simulink model "BG"  (R2014a)
settings: Solver=ode3  StartTime=0.0  StopTime=1  FixedStep=dt  MaxStep=dt  RelTol=1e-3
values from neighbouring files (symbols this model uses):
  a1 = .4    (= 0.4)    [parameters.m]
  a2 = .35    (= 0.35)    [parameters.m]
  a3 = .25    (= 0.25)    [parameters.m]
  aTc = 0.05    [parameters.m]
  dt = 1e-3    (= 0.001)    [parameters.m]
  g = 1    [parameters.m]
  K = 1    [parameters.m]
  mTc = 0.01    [parameters.m]
  OP1_0 = [ax1_0 ay1_0 0]    [parameters.m]
  OP2_0 = OP1_0 + P1P2_0    [parameters.m]
  OP3_0 = OP2_0 + P2P3_0    [parameters.m]
  OT = [xf yf 0]    [animation.m]    (also in parameters.m = [0.5 0.5 0])
  OT_cercle = [0.6 0.55 0]    [parameters.m]
  p1 = w2 + w3    (= 3)    [parameters.m]
  P1P2_0 = [ax2_0 ay2_0 0]    [parameters.m]
  p2 = w1 + w3    (= 4)    [parameters.m]
  P2P3_0 = [ax3_0 ay3_0 0]    [parameters.m]
  p3 = w2 + w1    (= 5)    [parameters.m]
  tau = 0.001    [parameters.m]
  theta1_0 = zero_vector    [parameters.m]
  theta2_0 = zero_vector    [parameters.m]
  theta3_0 = zero_vector    [parameters.m]
  Vmax = 30    [parameters.m]
  w1 = 3    [parameters.m]
  w2 = 2    [parameters.m]
  w3 = 1    [parameters.m]
  zero_vector = [0 0 0]    [parameters.m]
libraries: vrlib x9, simulink x1
(part 4 of 4)

== system BG/CNS/ Striosom//SNc2/Optimiseur/B2/Subsystem/matrix_by_matrix1 ==
  a11 : Inport
  a12 : Inport  Port=2
  a21 : Inport  Port=3
  a22 : Inport  Port=4
  b11 : Inport  Port=5
  b12 : Inport  Port=6
  b21 : Inport  Port=7
  b22 : Inport  Port=8
  "                                                                                                    " : Sum
  "                                                                                                     " : Sum
  "                                                                                                       " : Sum
  "                                                                                                          " : Sum
  a{1..8} (8 alike) : Product
  a11_out : Outport
  a12_out : Outport  Port=2
  a21_out : Outport  Port=3
  a22_out : Outport  Port=4
  wires:
  a11/1 -> a3/1, a1/1
  b11/1 -> a1/2, a5/2
  a12/1 -> a4/1, a2/1
  a1/1 -> "                                                                                                    "/1
  a2/1 -> "                                                                                                    "/2
  b21/1 -> a6/2, a2/2
  "                                                                                                    "/1 -> a11_out/1
  a3/1 -> "                                                                                                       "/1
  a4/1 -> "                                                                                                       "/2
  "                                                                                                       "/1 -> a12_out/1
  b22/1 -> a8/2, a4/2
  a21/1 -> a5/1, a7/1
  a5/1 -> "                                                                                                     "/1
  a6/1 -> "                                                                                                     "/2
  "                                                                                                     "/1 -> a21_out/1
  a7/1 -> "                                                                                                          "/1
  a8/1 -> "                                                                                                          "/2
  "                                                                                                          "/1 -> a22_out/1
  a22/1 -> a8/1, a6/1
  b12/1 -> a7/2, a3/2

== system BG/CNS/ Striosom//SNc2/Optimiseur/B2/Subsystem/vector_in_matrix_out1 ==
  v1 : Inport
  v2 : Inport  Port=2
  Demux : Demux  Outputs=3
  Demux1 : Demux  Outputs=3
  a{11..12,21..22} (4 alike) : Product
  a11_out : Outport
  a12_out : Outport  Port=2
  a21_out : Outport  Port=3
  a22_out : Outport  Port=4
  wires:
  v1/1 -> Demux/1
  v2/1 -> Demux1/1
  a11/1 -> a11_out/1
  Demux/1 -> a12/1, a11/1
  a12/1 -> a12_out/1
  a21/1 -> a21_out/1
  Demux/2 -> a22/1, a21/1
  a22/1 -> a22_out/1
  Demux1/1 -> a11/2, a21/2
  Demux1/2 -> a22/2, a12/2

== system BG/CNS/ Striosom//SNc2/Optimiseur/B2/Subsystem/vector_in_matrix_out2 ==
  v1 : Inport
  v2 : Inport  Port=2
  Demux : Demux  Outputs=3
  Demux1 : Demux  Outputs=3
  a{11..12,21..22} (4 alike) : Product
  a11_out : Outport
  a12_out : Outport  Port=2
  a21_out : Outport  Port=3
  a22_out : Outport  Port=4
  wires:
  v1/1 -> Demux/1
  v2/1 -> Demux1/1
  a11/1 -> a11_out/1
  Demux/1 -> a12/1, a11/1
  a12/1 -> a12_out/1
  a21/1 -> a21_out/1
  Demux/2 -> a22/1, a21/1
  a22/1 -> a22_out/1
  Demux1/1 -> a11/2, a21/2
  Demux1/2 -> a22/2, a12/2

== system BG/CNS/ Striosom//SNc2/Optimiseur/lambda/d=V^T(VV^T)^-1V/inverse_matrix ==
  a11 : Inport
  a12 : Inport  Port=2
  a21 : Inport  Port=3
  a22 : Inport  Port=4
  "                                                                                                    " : Sum  Inputs=+-+
  Divide{1..4} (4 alike) : Product  Inputs=*/
  Gain : Gain  Gain=-1
  Gain1 : Gain  Gain=-1
  a1 : Product
  a2 : Product
  eps : Constant  Value=1e-2
  a11_out : Outport
  a12_out : Outport  Port=2
  a21_out : Outport  Port=3
  a22_out : Outport  Port=4
  wires:
  a11/1 -> Divide2/1, a1/1
  a22/1 -> Divide1/1, a1/2
  a12/1 -> a2/1, Gain1/1
  a21/1 -> Gain/1, a2/2
  a1/1 -> "                                                                                                    "/1
  a2/1 -> "                                                                                                    "/2
  "                                                                                                    "/1 -> Divide1/2, Divide2/2, Divide3/2, Divide4/2
  Divide1/1 -> a11_out/1
  Divide2/1 -> a22_out/1
  Divide3/1 -> a12_out/1
  Divide4/1 -> a21_out/1
  Gain/1 -> Divide4/1
  Gain1/1 -> Divide3/1
  eps/1 -> "                                                                                                    "/3

== system BG/CNS/ Striosom//SNc2/Optimiseur/lambda/d=V^T(VV^T)^-1V/matrix_vector_multiplication ==
  a11 : Inport
  a12 : Inport  Port=2
  a21 : Inport  Port=3
  a22 : Inport  Port=4
  v1 : Inport  Port=5
  "                                                                                                    " : Sum
  "                                                                                                           " : Sum
  Demux : Demux  Outputs=3
  Mux : Mux  Inputs=3
  a{1..4} (4 alike) : Product
  vec_out : Outport
  wires:
  v1/1 -> Demux/1
  a11/1 -> a1/2
  a12/1 -> a2/2
  a1/1 -> "                                                                                                    "/1
  a2/1 -> "                                                                                                    "/2
  "                                                                                                    "/1 -> Mux/1
  Demux/1 -> a3/1, a1/1
  a21/1 -> a3/2
  Demux/2 -> a4/1, a2/1
  a22/1 -> a4/2
  a3/1 -> "                                                                                                           "/1
  a4/1 -> "                                                                                                           "/2
  "                                                                                                           "/1 -> Mux/2
  Mux/1 -> vec_out/1

== system BG/CNS/ Striosom//SNc2/Optimiseur/lambda/d=V^T(VV^T)^-1V/vector_in_matrix_out ==
  v1 : Inport
  v2 : Inport  Port=2
  Demux : Demux  Outputs=3
  Demux1 : Demux  Outputs=3
  a{11..12,21..22} (4 alike) : Product
  a11_out : Outport
  a12_out : Outport  Port=2
  a21_out : Outport  Port=3
  a22_out : Outport  Port=4
  wires:
  v1/1 -> Demux/1
  v2/1 -> Demux1/1
  a11/1 -> a11_out/1
  Demux/1 -> a12/1, a11/1
  a12/1 -> a12_out/1
  a21/1 -> a21_out/1
  Demux/2 -> a22/1, a21/1
  a22/1 -> a22_out/1
  Demux1/1 -> a11/2, a21/2
  Demux1/2 -> a22/2, a12/2

== system BG/CNS/ Striosom//SNc2/Optimiseur1/B1/Subsystem/matrix_by_matrix ==
  a11 : Inport
  a12 : Inport  Port=2
  a21 : Inport  Port=3
  a22 : Inport  Port=4
  b11 : Inport  Port=5
  b12 : Inport  Port=6
  b21 : Inport  Port=7
  b22 : Inport  Port=8
  "                                                                                                    " : Sum
  "                                                                                                     " : Sum
  "                                                                                                       " : Sum
  "                                                                                                          " : Sum
  a{1..8} (8 alike) : Product
  a11_out : Outport
  a12_out : Outport  Port=2
  a21_out : Outport  Port=3
  a22_out : Outport  Port=4
  wires:
  a11/1 -> a3/1, a1/1
  b11/1 -> a1/2, a5/2
  a12/1 -> a4/1, a2/1
  a1/1 -> "                                                                                                    "/1
  a2/1 -> "                                                                                                    "/2
  b21/1 -> a6/2, a2/2
  "                                                                                                    "/1 -> a11_out/1
  a3/1 -> "                                                                                                       "/1
  a4/1 -> "                                                                                                       "/2
  "                                                                                                       "/1 -> a12_out/1
  b22/1 -> a8/2, a4/2
  a21/1 -> a5/1, a7/1
  a5/1 -> "                                                                                                     "/1
  a6/1 -> "                                                                                                     "/2
  "                                                                                                     "/1 -> a21_out/1
  a7/1 -> "                                                                                                          "/1
  a8/1 -> "                                                                                                          "/2
  "                                                                                                          "/1 -> a22_out/1
  a22/1 -> a8/1, a6/1
  b12/1 -> a7/2, a3/2

== system BG/CNS/ Striosom//SNc2/Optimiseur1/B1/Subsystem/matrix_by_matrix1 ==
  a11 : Inport
  a12 : Inport  Port=2
  a21 : Inport  Port=3
  a22 : Inport  Port=4
  b11 : Inport  Port=5
  b12 : Inport  Port=6
  b21 : Inport  Port=7
  b22 : Inport  Port=8
  "                                                                                                    " : Sum
  "                                                                                                     " : Sum
  "                                                                                                       " : Sum
  "                                                                                                          " : Sum
  a{1..8} (8 alike) : Product
  a11_out : Outport
  a12_out : Outport  Port=2
  a21_out : Outport  Port=3
  a22_out : Outport  Port=4
  wires:
  a11/1 -> a3/1, a1/1
  b11/1 -> a1/2, a5/2
  a12/1 -> a4/1, a2/1
  a1/1 -> "                                                                                                    "/1
  a2/1 -> "                                                                                                    "/2
  b21/1 -> a6/2, a2/2
  "                                                                                                    "/1 -> a11_out/1
  a3/1 -> "                                                                                                       "/1
  a4/1 -> "                                                                                                       "/2
  "                                                                                                       "/1 -> a12_out/1
  b22/1 -> a8/2, a4/2
  a21/1 -> a5/1, a7/1
  a5/1 -> "                                                                                                     "/1
  a6/1 -> "                                                                                                     "/2
  "                                                                                                     "/1 -> a21_out/1
  a7/1 -> "                                                                                                          "/1
  a8/1 -> "                                                                                                          "/2
  "                                                                                                          "/1 -> a22_out/1
  a22/1 -> a8/1, a6/1
  b12/1 -> a7/2, a3/2

== system BG/CNS/ Striosom//SNc2/Optimiseur1/B1/Subsystem/vector_in_matrix_out1 ==
  v1 : Inport
  v2 : Inport  Port=2
  Demux : Demux  Outputs=3
  Demux1 : Demux  Outputs=3
  a{11..12,21..22} (4 alike) : Product
  a11_out : Outport
  a12_out : Outport  Port=2
  a21_out : Outport  Port=3
  a22_out : Outport  Port=4
  wires:
  v1/1 -> Demux/1
  v2/1 -> Demux1/1
  a11/1 -> a11_out/1
  Demux/1 -> a12/1, a11/1
  a12/1 -> a12_out/1
  a21/1 -> a21_out/1
  Demux/2 -> a22/1, a21/1
  a22/1 -> a22_out/1
  Demux1/1 -> a11/2, a21/2
  Demux1/2 -> a22/2, a12/2

== system BG/CNS/ Striosom//SNc2/Optimiseur1/B1/Subsystem/vector_in_matrix_out2 ==
  v1 : Inport
  v2 : Inport  Port=2
  Demux : Demux  Outputs=3
  Demux1 : Demux  Outputs=3
  a{11..12,21..22} (4 alike) : Product
  a11_out : Outport
  a12_out : Outport  Port=2
  a21_out : Outport  Port=3
  a22_out : Outport  Port=4
  wires:
  v1/1 -> Demux/1
  v2/1 -> Demux1/1
  a11/1 -> a11_out/1
  Demux/1 -> a12/1, a11/1
  a12/1 -> a12_out/1
  a21/1 -> a21_out/1
  Demux/2 -> a22/1, a21/1
  a22/1 -> a22_out/1
  Demux1/1 -> a11/2, a21/2
  Demux1/2 -> a22/2, a12/2

== system BG/CNS/ Striosom//SNc2/Optimiseur1/B2/Subsystem/matrix_by_matrix ==
  a11 : Inport
  a12 : Inport  Port=2
  a21 : Inport  Port=3
  a22 : Inport  Port=4
  b11 : Inport  Port=5
  b12 : Inport  Port=6
  b21 : Inport  Port=7
  b22 : Inport  Port=8
  "                                                                                                    " : Sum
  "                                                                                                     " : Sum
  "                                                                                                       " : Sum
  "                                                                                                          " : Sum
  a{1..8} (8 alike) : Product
  a11_out : Outport
  a12_out : Outport  Port=2
  a21_out : Outport  Port=3
  a22_out : Outport  Port=4
  wires:
  a11/1 -> a3/1, a1/1
  b11/1 -> a1/2, a5/2
  a12/1 -> a4/1, a2/1
  a1/1 -> "                                                                                                    "/1
  a2/1 -> "                                                                                                    "/2
  b21/1 -> a6/2, a2/2
  "                                                                                                    "/1 -> a11_out/1
  a3/1 -> "                                                                                                       "/1
  a4/1 -> "                                                                                                       "/2
  "                                                                                                       "/1 -> a12_out/1
  b22/1 -> a8/2, a4/2
  a21/1 -> a5/1, a7/1
  a5/1 -> "                                                                                                     "/1
  a6/1 -> "                                                                                                     "/2
  "                                                                                                     "/1 -> a21_out/1
  a7/1 -> "                                                                                                          "/1
  a8/1 -> "                                                                                                          "/2
  "                                                                                                          "/1 -> a22_out/1
  a22/1 -> a8/1, a6/1
  b12/1 -> a7/2, a3/2

== system BG/CNS/ Striosom//SNc2/Optimiseur1/B2/Subsystem/matrix_by_matrix1 ==
  a11 : Inport
  a12 : Inport  Port=2
  a21 : Inport  Port=3
  a22 : Inport  Port=4
  b11 : Inport  Port=5
  b12 : Inport  Port=6
  b21 : Inport  Port=7
  b22 : Inport  Port=8
  "                                                                                                    " : Sum
  "                                                                                                     " : Sum
  "                                                                                                       " : Sum
  "                                                                                                          " : Sum
  a{1..8} (8 alike) : Product
  a11_out : Outport
  a12_out : Outport  Port=2
  a21_out : Outport  Port=3
  a22_out : Outport  Port=4
  wires:
  a11/1 -> a3/1, a1/1
  b11/1 -> a1/2, a5/2
  a12/1 -> a4/1, a2/1
  a1/1 -> "                                                                                                    "/1
  a2/1 -> "                                                                                                    "/2
  b21/1 -> a6/2, a2/2
  "                                                                                                    "/1 -> a11_out/1
  a3/1 -> "                                                                                                       "/1
  a4/1 -> "                                                                                                       "/2
  "                                                                                                       "/1 -> a12_out/1
  b22/1 -> a8/2, a4/2
  a21/1 -> a5/1, a7/1
  a5/1 -> "                                                                                                     "/1
  a6/1 -> "                                                                                                     "/2
  "                                                                                                     "/1 -> a21_out/1
  a7/1 -> "                                                                                                          "/1
  a8/1 -> "                                                                                                          "/2
  "                                                                                                          "/1 -> a22_out/1
  a22/1 -> a8/1, a6/1
  b12/1 -> a7/2, a3/2

== system BG/CNS/ Striosom//SNc2/Optimiseur1/B2/Subsystem/vector_in_matrix_out1 ==
  v1 : Inport
  v2 : Inport  Port=2
  Demux : Demux  Outputs=3
  Demux1 : Demux  Outputs=3
  a{11..12,21..22} (4 alike) : Product
  a11_out : Outport
  a12_out : Outport  Port=2
  a21_out : Outport  Port=3
  a22_out : Outport  Port=4
  wires:
  v1/1 -> Demux/1
  v2/1 -> Demux1/1
  a11/1 -> a11_out/1
  Demux/1 -> a12/1, a11/1
  a12/1 -> a12_out/1
  a21/1 -> a21_out/1
  Demux/2 -> a22/1, a21/1
  a22/1 -> a22_out/1
  Demux1/1 -> a11/2, a21/2
  Demux1/2 -> a22/2, a12/2

== system BG/CNS/ Striosom//SNc2/Optimiseur1/B2/Subsystem/vector_in_matrix_out2 ==
  v1 : Inport
  v2 : Inport  Port=2
  Demux : Demux  Outputs=3
  Demux1 : Demux  Outputs=3
  a{11..12,21..22} (4 alike) : Product
  a11_out : Outport
  a12_out : Outport  Port=2
  a21_out : Outport  Port=3
  a22_out : Outport  Port=4
  wires:
  v1/1 -> Demux/1
  v2/1 -> Demux1/1
  a11/1 -> a11_out/1
  Demux/1 -> a12/1, a11/1
  a12/1 -> a12_out/1
  a21/1 -> a21_out/1
  Demux/2 -> a22/1, a21/1
  a22/1 -> a22_out/1
  Demux1/1 -> a11/2, a21/2
  Demux1/2 -> a22/2, a12/2

== system BG/CNS/ Striosom//SNc2/Optimiseur1/lambda/d=V^T(VV^T)^-1V/inverse_matrix ==
  a11 : Inport
  a12 : Inport  Port=2
  a21 : Inport  Port=3
  a22 : Inport  Port=4
  "                                                                                                    " : Sum  Inputs=+-+
  Divide{1..4} (4 alike) : Product  Inputs=*/
  Gain : Gain  Gain=-1
  Gain1 : Gain  Gain=-1
  a1 : Product
  a2 : Product
  eps : Constant  Value=1e-3
  a11_out : Outport
  a12_out : Outport  Port=2
  a21_out : Outport  Port=3
  a22_out : Outport  Port=4
  wires:
  a11/1 -> Divide2/1, a1/1
  a22/1 -> Divide1/1, a1/2
  a12/1 -> a2/1, Gain1/1
  a21/1 -> Gain/1, a2/2
  a1/1 -> "                                                                                                    "/1
  a2/1 -> "                                                                                                    "/2
  "                                                                                                    "/1 -> Divide1/2, Divide2/2, Divide3/2, Divide4/2
  Divide1/1 -> a11_out/1
  Divide2/1 -> a22_out/1
  Divide3/1 -> a12_out/1
  Divide4/1 -> a21_out/1
  Gain/1 -> Divide4/1
  Gain1/1 -> Divide3/1
  eps/1 -> "                                                                                                    "/3

== system BG/CNS/ Striosom//SNc2/Optimiseur1/lambda/d=V^T(VV^T)^-1V/matrix_vector_multiplication ==
  a11 : Inport
  a12 : Inport  Port=2
  a21 : Inport  Port=3
  a22 : Inport  Port=4
  v1 : Inport  Port=5
  "                                                                                                    " : Sum
  "                                                                                                           " : Sum
  Demux : Demux  Outputs=3
  Mux : Mux  Inputs=3
  a{1..4} (4 alike) : Product
  vec_out : Outport
  wires:
  v1/1 -> Demux/1
  a11/1 -> a1/2
  a12/1 -> a2/2
  a1/1 -> "                                                                                                    "/1
  a2/1 -> "                                                                                                    "/2
  "                                                                                                    "/1 -> Mux/1
  Demux/1 -> a3/1, a1/1
  a21/1 -> a3/2
  Demux/2 -> a4/1, a2/1
  a22/1 -> a4/2
  a3/1 -> "                                                                                                           "/1
  a4/1 -> "                                                                                                           "/2
  "                                                                                                           "/1 -> Mux/2
  Mux/1 -> vec_out/1

== system BG/CNS/ Striosom//SNc2/Optimiseur1/lambda/d=V^T(VV^T)^-1V/vector_in_matrix_out ==
  v1 : Inport
  v2 : Inport  Port=2
  Demux : Demux  Outputs=3
  Demux1 : Demux  Outputs=3
  a{11..12,21..22} (4 alike) : Product
  a11_out : Outport
  a12_out : Outport  Port=2
  a21_out : Outport  Port=3
  a22_out : Outport  Port=4
  wires:
  v1/1 -> Demux/1
  v2/1 -> Demux1/1
  a11/1 -> a11_out/1
  Demux/1 -> a12/1, a11/1
  a12/1 -> a12_out/1
  a21/1 -> a21_out/1
  Demux/2 -> a22/1, a21/1
  a22/1 -> a22_out/1
  Demux1/1 -> a11/2, a21/2
  Demux1/2 -> a22/2, a12/2
